simulink model "PWM_Model"  (R2019b)
settings: Solver=VariableStepAuto  StartTime=0.0  StopTime=10.0  RelTol=1e-3
model workspace (MAT data in the model file):
  MCU_freq = Simulink.Parameter
  MCU_freq.Value = 1000000
  MCU_freq.DataType = 'auto'
  MCU_freq.Dimensions = [1 1]
  MCU_timerDesiredFreq = Simulink.Parameter
  MCU_timerDesiredFreq.Value = 50
  MCU_timerDesiredFreq.DataType = 'auto'
  MCU_timerDesiredFreq.Dimensions = [1 1]
  MCU_timerPrescaler = Simulink.Parameter
  MCU_timerPrescaler.Value = 16
  MCU_timerPrescaler.DataType = 'auto'
  MCU_timerPrescaler.Dimensions = [1 1]
  Servo_PWM_0_degree = Simulink.Parameter
  Servo_PWM_0_degree.Value = 4.5
  Servo_PWM_0_degree.DataType = 'auto'
  Servo_PWM_0_degree.Dimensions = [1 1]
  Servo_PWM_180_degree = Simulink.Parameter
  Servo_PWM_180_degree.Value = 10.5
  Servo_PWM_180_degree.DataType = 'auto'
  Servo_PWM_180_degree.Dimensions = [1 1]
undefined symbols (not defined in the file): m, n, sigbuilder_block
libraries: aerolibanimutils x1
settings Model: OrderedModelArguments=off  Creator=OBU  LastModifiedBy=toons

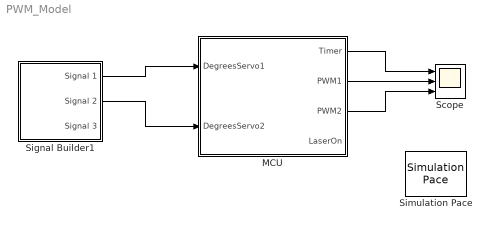
== system PWM_Model ==
  MCU : Subsystem
  Scope : Scope  NumInputPorts=3
  Signal Builder1 : Subsystem  Tag=STV Subsys  LoadFcn=sigbuilder_block('load');  StartFcn=sigbuilder_block('start');  StopFcn=sigbuilder_block('stop');  ClipboardFcn=sigbuilder_block('clipboard');  mask(Sigbuilder block){tuvar=[0:10]}
      mask help: Simulink:masks:SigbuilderBlock_MD
      mask init:
      | if ~strcmp(get_param(bdroot(gcbh),'SimulationStatus'),'stopped') tuvar = sigbuilder_block('maskInit'); end
      settings: CopyFcn=sigbuilder_block('copy');  DeleteFcn=sigbuilder_block('delete');  ModelCloseFcn=sigbuilder_block('modelClose');  PreSaveFcn=sigbuilder_block('preSave');  PauseFcn=sigbuilder_block('pause');  ContinueFcn=sigbuilder_block('continue');  NameChangeFcn=sigbuilder_block('namechange');  OpenFcn=sigbuilder_block('open',[355.2 161.4 550.8 400.2 ]);  CloseFcn=sigbuilder_block('close');
      mask Display: plot(0, 0, 100, 100,[2, 2, 32, 32, 2], [68, 8, 8, 68, 68],[32, 2], [38, 38], [32, 19, 2],[53, 60, 44], [32, 17, 17, 2],[16, 16, 31, 31]);txt = getActiveGroup(gcbh);text(2, 100, txt,'verticalAlignment', 'top');
  Simulation Pace : aerolibanimutils/Simulation Pace  SimulationPace=1  SleepMode=Auto  OutputPaceError=off  SampleTime=1/30
  wires:
  Signal Builder1/1(Signal 1) -> MCU/1("DegreesServo1 ")
  Signal Builder1/2(Signal 2) -> MCU/2(DegreesServo2)
  MCU/2("PWM1 ") -> Scope/2
  MCU/3(PWM2) -> Scope/3
  MCU/1(Timer) -> Scope/1

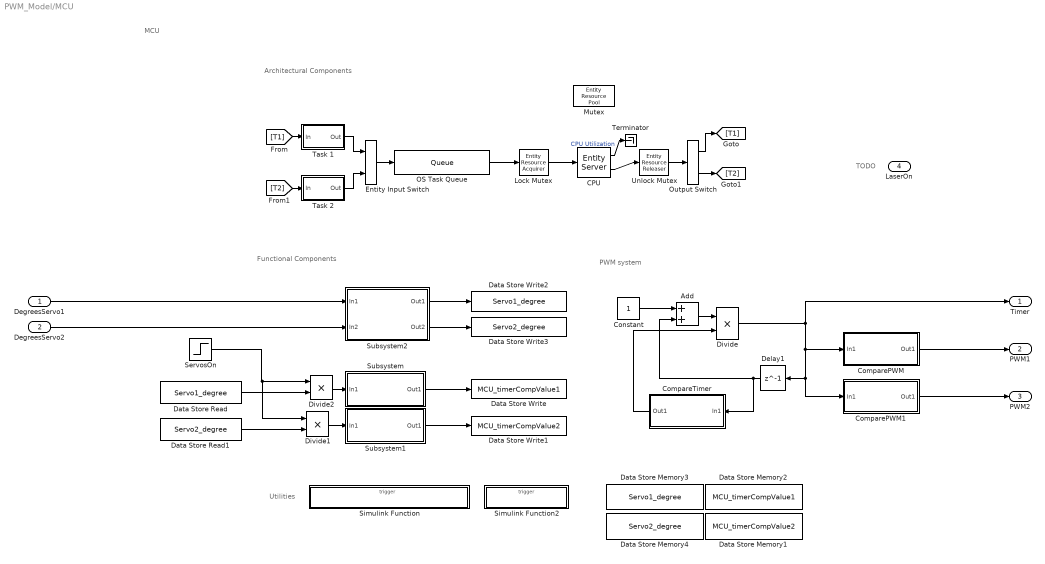
== system PWM_Model/MCU ==
  note: TODO
  note: PWM system
  note: MCU
  note: Functional Components
  note: Utilities
  note: Architectural Components
  "DegreesServo1 " : Inport
  DegreesServo2 : Inport  Port=2
  Add : Sum
  CPU : EntityServer  InputPortMessageModes=m  OutputPortMessageModes=n,m  Capacity=1  ServiceTimeSource=MATLAB action  ServiceTimeAttributeName=remExecLoad  ServiceTimeAction=dt = entity.execLoad(entity.nextSegment);  EntryAction=|  ServiceCompleteAction=|  ExitAction=|  SortingAttributeName=taskPriority  WriteResidualTimeToAttribute=on  ResidualTimeAttributeName=remExecLoad  Utilization=on
      EntryAction=|
      | start = 0;
      | entity.coreID = allocCore(start);
      | numSegments = length(entity.execLoad);
      | drawTaskTiming(entity.taskID, ...
      |                entity.nextSegment, ...
      |                numSegments, ...
      |                entity.coreID, ...
      |                entity.needsMutexForNextSegment, ...
      |                start);
      ServiceCompleteAction=|
      | switch entity.taskID
      |     case 1
      |         switch entity.nextSegment
      |             case 1
      |                 servo1_set_degree();
      |             case 2
      |                 servo2_set_degree();
      |         end
      |     case 2
      |         switch entity.nextSegment
      |             case 1
      |                 pwm1_set();
      |             case 2
      |                 pwm2_set();
      |         end
      | end
      ExitAction=|
      | complete = 1;
      | numSegments = length(entity.execLoad);
      | drawTaskTiming(entity.taskID, ...
      |                entity.nextSegment, ...
      |                numSegments, ...
      |                entity.coreID, ...
      |                entity.needsMutexForNextSegment, ...
      |                complete);
      | allocCore(entity.coreID);
      settings: OutputPortMap=o5,o9
  ComparePWM : Subsystem
  ComparePWM1 : Subsystem
  CompareTimer : Subsystem
  Constant : Constant
  Data Store Memory1 : DataStoreMemory  DataStoreName=MCU_timerCompValue2  ReadBeforeWriteMsg=warning  WriteAfterWriteMsg=warning  WriteAfterReadMsg=warning  InitialValue=400  ShowAdditionalParam=off  OutDataTypeStr=double
  Data Store Memory2 : DataStoreMemory  DataStoreName=MCU_timerCompValue1  ReadBeforeWriteMsg=warning  WriteAfterWriteMsg=warning  WriteAfterReadMsg=warning  InitialValue=400  ShowAdditionalParam=off  OutDataTypeStr=double
  Data Store Memory3 : DataStoreMemory  DataStoreName=Servo1_degree  ReadBeforeWriteMsg=warning  WriteAfterWriteMsg=warning  WriteAfterReadMsg=warning  InitialValue=400  ShowAdditionalParam=off  OutDataTypeStr=double
  Data Store Memory4 : DataStoreMemory  DataStoreName=Servo2_degree  ReadBeforeWriteMsg=warning  WriteAfterWriteMsg=warning  WriteAfterReadMsg=warning  InitialValue=400  ShowAdditionalParam=off  OutDataTypeStr=double
  Data Store Read : DataStoreRead  DataStoreName=Servo1_degree
  Data Store Read1 : DataStoreRead  DataStoreName=Servo2_degree
  Data Store Write : DataStoreWrite  DataStoreName=MCU_timerCompValue1
  Data Store Write1 : DataStoreWrite  DataStoreName=MCU_timerCompValue2
  Data Store Write2 : DataStoreWrite  DataStoreName=Servo1_degree
  Data Store Write3 : DataStoreWrite  DataStoreName=Servo2_degree
  Delay1 : Delay  DelayLength=1  SampleTime=1/(MCU_freq/MCU_timerPrescaler)
  Divide : Product  Inputs=**  SaturateOnIntegerOverflow=on  RndMeth=Zero
  Divide1 : Product  Inputs=**  SaturateOnIntegerOverflow=on  RndMeth=Zero
  Divide2 : Product  Inputs=**  SaturateOnIntegerOverflow=on  RndMeth=Zero
  Entity Input Switch : EntityInputSwitch  InputPortMessageModes=m,m  OutputPortMessageModes=m
  Lock Mutex : EntityResourceAcquirer  InputPortMessageModes=m  OutputPortMessageModes=m  EntryAction=entity.needsMutexForNextSegment = entity.needsResource(entity.nextSegment);  ResourceName=DiskLock  ResourceAmountSource=Attribute  ResourceAmount=needsMutexForNextSegment
      settings: OutputPortMap=o3
  Mutex : EntityResourcePool  ResourceName=DiskLock  ResourceAmount=1
  OS Task Queue : Queue  InputPortMessageModes=m  OutputPortMessageModes=m  Capacity=100  QueueType=Priority  PrioritySource=taskPriority  MulticastTag=TaskReady
  Output Switch : EntityOutputSwitch  InputPortMessageModes=m  OutputPortMessageModes=m,m  SwitchingCriterion=From attribute  SwitchAttributeName=taskID
  ServosOn : Step  SampleTime=0
  Simulink Function : Subsystem  TreatAsAtomicUnit=on
  Simulink Function2 : Subsystem  TreatAsAtomicUnit=on
  Subsystem : Subsystem
  Subsystem1 : Subsystem
  Subsystem2 : Subsystem
  Task 1 : Subsystem  mask{taskID=1, period=0.5, taskPriority=100, taskFunction=servo1_set_degree, servo2_set_degree, execLoad=[0.1, 0.1], needsResource=[0 0]}
      mask prompts: taskID "ID:"; taskPriority "Priority:"; taskFunction "List of runnable segments (functions):"; execLoad "Segment execution load vector:"; needsResource "Needs disk i/o resource for each segment:"
      mask DialogControl DescGroupVar Prompt: OS Task
      mask DialogControl DescTextVar Prompt: Model and simulate a task of a real-time operating system.
      mask Display: disp(['Task ' get_param(gcb, 'taskID')])
  Task 2 : Subsystem  mask{taskID=2, period=0.5, taskPriority=50, execLoad=[0.1, 0.1], taskFunction=pwm1_set,pwm2_set, needsResource=[0 0]}
      mask prompts: taskID "ID:"; taskPriority "Priority:"; execLoad "Segment execution load vector:"; taskFunction "List of runnable segments (functions):"; needsResource "Needs disk i/o resource for each segment:"
      mask DialogControl DescGroupVar Prompt: OS Task
      mask DialogControl DescTextVar Prompt: Model and simulate a task of a real-time operating system.
      mask Display: disp(['Task ' get_param(gcb, 'taskID')])
  Terminator : Terminator
  Unlock Mutex : EntityResourceReleaser  InputPortMessageModes=m  OutputPortMessageModes=m
  Timer : Outport
  "PWM1 " : Outport  Port=2
  PWM2 : Outport  Port=3
  LaserOn : Outport  Port=4
  wires:
  Task 1/1(Out) -> Entity Input Switch/1
  Divide/1 -> Timer/1, ComparePWM1/1(In1), Delay1/1, ComparePWM/1(In1)
  Entity Input Switch/1 -> OS Task Queue/1
  [T2] -> Task 2/1(In)
  Lock Mutex/1 -> CPU/1
  Task 2/1(Out) -> Entity Input Switch/2
  Output Switch/1 -> [T1]
  Unlock Mutex/1 -> Output Switch/1
  CPU/2 -> Unlock Mutex/1
  OS Task Queue/1 -> Lock Mutex/1
  Constant/1 -> Add/1
  CompareTimer/1(Out1) -> Divide/2
  Delay1/1 -> Add/2, CompareTimer/1(In1)
  Add/1 -> Divide/1
  [T1] -> Task 1/1(In)
  CPU/1 -> Terminator/1  "CPU Utilization"
  Output Switch/2 -> [T2]
  DegreesServo2/1 -> Subsystem2/2(In2)
  "DegreesServo1 "/1 -> Subsystem2/1(In1)
  ComparePWM/1(Out1) -> "PWM1 "/1
  ComparePWM1/1(Out1) -> PWM2/1
  Subsystem1/1(Out1) -> Data Store Write1/1
  Subsystem/1(Out1) -> Data Store Write/1
  Subsystem2/1(Out1) -> Data Store Write2/1
  Subsystem2/2(Out2) -> Data Store Write3/1
  Divide2/1 -> Subsystem/1(In1)
  Data Store Read/1 -> Divide2/2
  Divide1/1 -> Subsystem1/1(In1)
  ServosOn/1 -> Divide1/1, Divide2/1
  Data Store Read1/1 -> Divide1/2

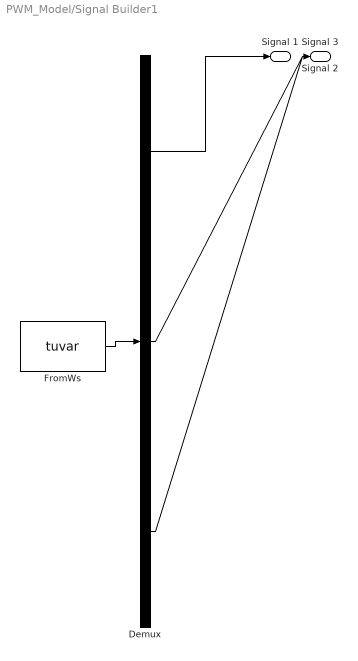
== system PWM_Model/Signal Builder1 ==
  Demux : Demux  Tag=STV Demux  Outputs=3
  FromWs : FromWorkspace  Tag=STV FromWs  VariableName=tuvar  SampleTime=0
      SigBuilderData=|
      | common.afterFinalStr = 'Extrapolate'
      | common.sampleTime = 0
      | dataSet.timeRange = [0 10]
      | dataSet.name = 'Group 1'
      | sbobj.Groups.Name = 'Group 1'
      | sbobj.Groups.Signals(1).Name = 'Signal 1'
      | sbobj.Groups.Signals(1).XData = [0 4 5 6 10]
      | sbobj.Groups.Signals(1).YData = [0 180 90 90 0]
      | sbobj.Groups.Signals(2).Name = 'Signal 2'
      | sbobj.Groups.Signals(2).XData = [0 2 5 10]
      | sbobj.Groups.Signals(2).YData = [0 0 180 180]
      | sbobj.Groups.Signals(3).Name = 'Signal 3'
      | sbobj.Groups.Signals(3).XData = [0 4 4 6 6 10]
      | sbobj.Groups.Signals(3).YData = [0 0 1 1 0 0]
  Signal 1 : Outport  Tag=STV Outport
  Signal 2 : Outport  Tag=STV Outport  Port=2
  Signal 3 : Outport  Tag=STV Outport  Port=3
  wires:
  Demux/1 -> Signal 1/1
  FromWs/1 -> Demux/1
  Demux/2 -> Signal 2/1
  Demux/3 -> Signal 3/1

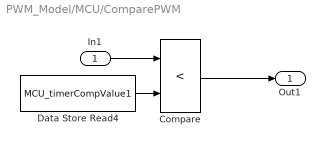
== system PWM_Model/MCU/ComparePWM ==
  In1 : Inport
  Compare : RelationalOperator  Operator=<  OutDataTypeStr=boolean  RndMeth=Nearest  InputSameDT=on
  Data Store Read4 : DataStoreRead  DataStoreName=MCU_timerCompValue1
  Out1 : Outport
  wires:
  In1/1 -> Compare/1
  Compare/1 -> Out1/1
  Data Store Read4/1 -> Compare/2

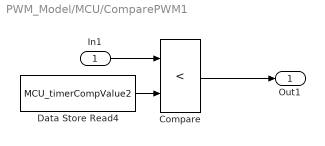
== system PWM_Model/MCU/ComparePWM1 ==
  In1 : Inport
  Compare : RelationalOperator  Operator=<  OutDataTypeStr=boolean  RndMeth=Nearest  InputSameDT=on
  Data Store Read4 : DataStoreRead  DataStoreName=MCU_timerCompValue2
  Out1 : Outport
  wires:
  In1/1 -> Compare/1
  Compare/1 -> Out1/1
  Data Store Read4/1 -> Compare/2

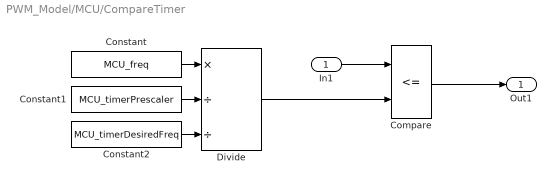
== system PWM_Model/MCU/CompareTimer ==
  In1 : Inport
  Compare : RelationalOperator  Operator=<=  OutDataTypeStr=boolean  RndMeth=Nearest  InputSameDT=on
  Constant : Constant  Value=MCU_freq
  Constant1 : Constant  Value=MCU_timerPrescaler
  Constant2 : Constant  Value=MCU_timerDesiredFreq
  Divide : Product  Inputs=*//
  Out1 : Outport
  wires:
  Compare/1 -> Out1/1
  Constant2/1 -> Divide/3
  Constant1/1 -> Divide/2
  Constant/1 -> Divide/1
  Divide/1 -> Compare/2
  In1/1 -> Compare/1

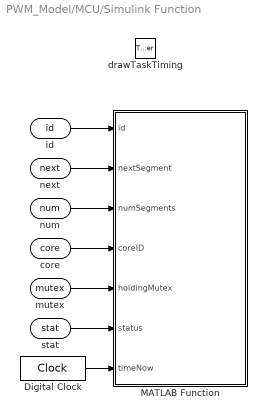
== system PWM_Model/MCU/Simulink Function ==
  drawTaskTiming : TriggerPort  TriggerType=function-call  IsSimulinkFunction=on  FunctionName=drawTaskTiming  VariantControl=Variant
  Digital Clock : DigitalClock  SampleTime=-1
  MATLAB Function : MATLAB Function  TreatAsAtomicUnit=on
  id : ArgIn  DisableCoverage=on  ArgumentName=id
  next : ArgIn  Port=2  ArgumentName=next
  num : ArgIn  Port=3  ArgumentName=num
  core : ArgIn  Port=4  ArgumentName=core
  mutex : ArgIn  Port=5  ArgumentName=mutex
  stat : ArgIn  Port=6  ArgumentName=stat
  wires:
  id/1 -> MATLAB Function/1(id)
  next/1 -> MATLAB Function/2(nextSegment)
  num/1 -> MATLAB Function/3(numSegments)
  Digital Clock/1 -> MATLAB Function/7(timeNow)
  core/1 -> MATLAB Function/4(coreID)
  mutex/1 -> MATLAB Function/5(holdingMutex)
  stat/1 -> MATLAB Function/6(status)

== system PWM_Model/MCU/Simulink Function2 ==
  allocCore : TriggerPort  TriggerType=function-call  IsSimulinkFunction=on  FunctionName=allocCore  VariantControl=Variant
  MATLAB Function : MATLAB Function  TreatAsAtomicUnit=on
  status : ArgIn  ArgumentName=status
  id : ArgOut  ArgumentName=id
  wires:
  status/1 -> MATLAB Function/1(status)
  MATLAB Function/1(id) -> id/1

== system PWM_Model/MCU/Subsystem ==
  In1 : Inport
  Subsystem : Subsystem
  Out1 : Outport
  wires:
  In1/1 -> Subsystem/1(In1)
  Subsystem/1(Out1) -> Out1/1

== system PWM_Model/MCU/Subsystem1 ==
  In1 : Inport
  Subsystem : Subsystem
  Out1 : Outport
  wires:
  In1/1 -> Subsystem/1(In1)
  Subsystem/1(Out1) -> Out1/1

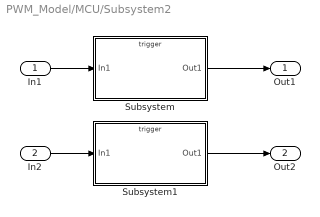
== system PWM_Model/MCU/Subsystem2 ==
  In1 : Inport
  In2 : Inport  Port=2
  Subsystem : Subsystem
  Subsystem1 : Subsystem
  Out1 : Outport
  Out2 : Outport  Port=2
  wires:
  In1/1 -> Subsystem/1(In1)
  Subsystem/1(Out1) -> Out1/1
  Subsystem1/1(Out1) -> Out2/1
  In2/1 -> Subsystem1/1(In1)

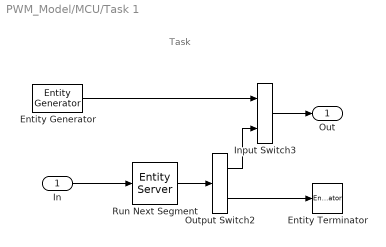
== system PWM_Model/MCU/Task 1 ==
  note: Task
  In : Inport
  Entity Generator : EntityGenerator  OutputPortMessageModes=m  Period=period  AttributeName=period|numSegments|execLoad|taskPriority|taskID|nextSegment|complete|coreID|needsMutexForNextSegment|needsResource  AttributeInitialValue=period|length(execLoad)|[execLoad zeros(1,20-length(execLoad))]|taskPriority|taskID|1|1|-1|0|[needsResource zeros(1,100-length(needsResource))]  EntityType=Structured  EntityTypeName=Task  EntityPriority=taskPriority
  Entity Terminator : EntityTerminator  InputPortMessageModes=m
  Input Switch3 : EntityInputSwitch  InputPortMessageModes=m,m  OutputPortMessageModes=m
  Output Switch2 : EntityOutputSwitch  InputPortMessageModes=m  OutputPortMessageModes=m,m  SwitchingCriterion=From attribute  SwitchAttributeName=complete
  Run Next Segment : EntityServer  InputPortMessageModes=m  OutputPortMessageModes=m  Capacity=1  ServiceTimeValue=0  ServiceCompleteAction=|
      | entity.nextSegment=entity.nextSegment+1;
      | if entity.nextSegment>entity.numSegments
      |     entity.complete=2;
      | else
      |     entity.needsMutexForNextSegment=entity.needsResource(entity.nextSegment);
      | end
  Out : Outport  VectorParamsAs1DForOutWhenUnconnected=off
  wires:
  In/1 -> Run Next Segment/1
  Entity Generator/1 -> Input Switch3/1
  Input Switch3/1 -> Out/1
  Run Next Segment/1 -> Output Switch2/1
  Output Switch2/1 -> Input Switch3/2
  Output Switch2/2 -> Entity Terminator/1

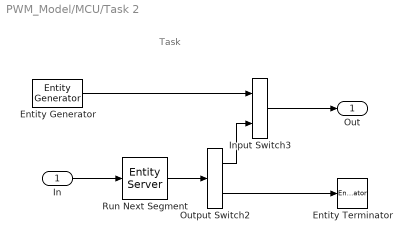
== system PWM_Model/MCU/Task 2 ==
  note: Task
  In : Inport
  Entity Generator : EntityGenerator  OutputPortMessageModes=m  Period=period  AttributeName=period|numSegments|execLoad|taskPriority|taskID|nextSegment|complete|coreID|needsMutexForNextSegment|needsResource  AttributeInitialValue=period|length(execLoad)|[execLoad zeros(1,20-length(execLoad))]|taskPriority|taskID|1|1|-1|0|[needsResource zeros(1,100-length(needsResource))]  EntityType=Structured  EntityTypeName=Task  EntityPriority=taskPriority
  Entity Terminator : EntityTerminator  InputPortMessageModes=m
  Input Switch3 : EntityInputSwitch  InputPortMessageModes=m,m  OutputPortMessageModes=m
  Output Switch2 : EntityOutputSwitch  InputPortMessageModes=m  OutputPortMessageModes=m,m  SwitchingCriterion=From attribute  SwitchAttributeName=complete
  Run Next Segment : EntityServer  InputPortMessageModes=m  OutputPortMessageModes=m  Capacity=1  ServiceTimeValue=0  ServiceCompleteAction=|
      | entity.nextSegment=entity.nextSegment+1;
      | if entity.nextSegment>entity.numSegments
      |     entity.complete=2;
      | else
      |     entity.needsMutexForNextSegment=entity.needsResource(entity.nextSegment);    
      | end
  Out : Outport  VectorParamsAs1DForOutWhenUnconnected=off
  wires:
  In/1 -> Run Next Segment/1
  Entity Generator/1 -> Input Switch3/1
  Input Switch3/1 -> Out/1
  Run Next Segment/1 -> Output Switch2/1
  Output Switch2/1 -> Input Switch3/2
  Output Switch2/2 -> Entity Terminator/1

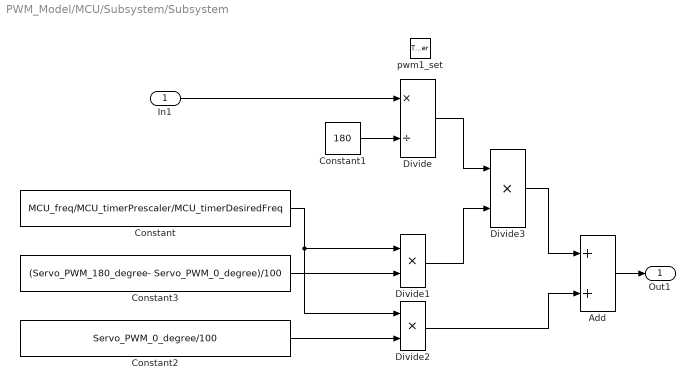
== system PWM_Model/MCU/Subsystem/Subsystem ==
  In1 : Inport
  pwm1_set : TriggerPort  TriggerType=function-call  IsSimulinkFunction=on  FunctionName=pwm1_set  VariantControl=Variant
  Add : Sum
  Constant : Constant  Value=MCU_freq/MCU_timerPrescaler/MCU_timerDesiredFreq
  Constant1 : Constant  Value=180
  Constant2 : Constant  Value=Servo_PWM_0_degree/100
  Constant3 : Constant  Value=(Servo_PWM_180_degree- Servo_PWM_0_degree)/100
  Divide : Product  Inputs=*/  SaturateOnIntegerOverflow=on  RndMeth=Zero
  Divide1 : Product  Inputs=**  SaturateOnIntegerOverflow=on  RndMeth=Zero
  Divide2 : Product  Inputs=**  SaturateOnIntegerOverflow=on  RndMeth=Zero
  Divide3 : Product  Inputs=**  SaturateOnIntegerOverflow=on  RndMeth=Zero
  Out1 : Outport
  wires:
  Constant1/1 -> Divide/2
  Constant/1 -> Divide1/1, Divide2/1
  Constant2/1 -> Divide2/2
  Constant3/1 -> Divide1/2
  Divide/1 -> Divide3/1
  Divide1/1 -> Divide3/2
  Divide2/1 -> Add/2
  Divide3/1 -> Add/1
  In1/1 -> Divide/1
  Add/1 -> Out1/1

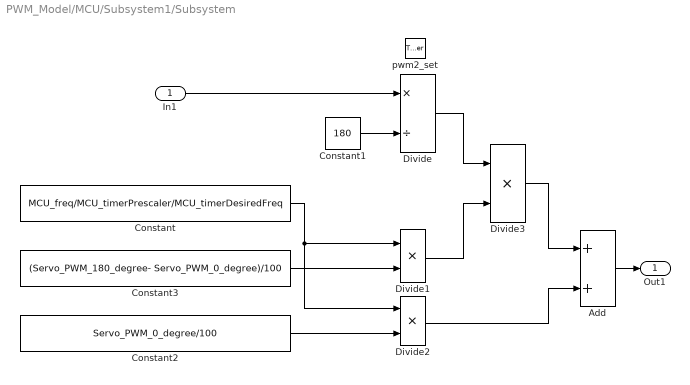
== system PWM_Model/MCU/Subsystem1/Subsystem ==
  In1 : Inport
  pwm2_set : TriggerPort  TriggerType=function-call  IsSimulinkFunction=on  FunctionName=pwm2_set  VariantControl=Variant
  Add : Sum
  Constant : Constant  Value=MCU_freq/MCU_timerPrescaler/MCU_timerDesiredFreq
  Constant1 : Constant  Value=180
  Constant2 : Constant  Value=Servo_PWM_0_degree/100
  Constant3 : Constant  Value=(Servo_PWM_180_degree- Servo_PWM_0_degree)/100
  Divide : Product  Inputs=*/  SaturateOnIntegerOverflow=on  RndMeth=Zero
  Divide1 : Product  Inputs=**  SaturateOnIntegerOverflow=on  RndMeth=Zero
  Divide2 : Product  Inputs=**  SaturateOnIntegerOverflow=on  RndMeth=Zero
  Divide3 : Product  Inputs=**  SaturateOnIntegerOverflow=on  RndMeth=Zero
  Out1 : Outport
  wires:
  Constant1/1 -> Divide/2
  Constant3/1 -> Divide1/2
  Divide2/1 -> Add/2
  Divide/1 -> Divide3/1
  In1/1 -> Divide/1
  Constant/1 -> Divide1/1, Divide2/1
  Add/1 -> Out1/1
  Constant2/1 -> Divide2/2
  Divide3/1 -> Add/1
  Divide1/1 -> Divide3/2

== system PWM_Model/MCU/Subsystem2/Subsystem ==
  In1 : Inport
  servo1_set_degree : TriggerPort  TriggerType=function-call  IsSimulinkFunction=on  FunctionName=servo1_set_degree  VariantControl=Variant
  Out1 : Outport
  wires:
  In1/1 -> Out1/1

== system PWM_Model/MCU/Subsystem2/Subsystem1 ==
  In1 : Inport
  servo2_set_degree : TriggerPort  TriggerType=function-call  IsSimulinkFunction=on  FunctionName=servo2_set_degree  VariantControl=Variant
  Out1 : Outport
  wires:
  In1/1 -> Out1/1

== matlab function PWM_Model/MCU/Simulink Function2/MATLAB Function ==
  data: status input; id output
function id = allocCore(status)
%#codegen

persistent allocCores
if isempty(allocCores)
    allocCores = zeros(1,100);
end

id = -1;

if status == 0
    for i = 1:100
        if allocCores(i) == 0
            id = i;
            allocCores(i) = 1;
            break;
        end
    end
else
    allocCores(status) = 0;
end

== matlab function PWM_Model/MCU/Simulink Function/MATLAB Function ==
  data: id input; nextSegment input; numSegments input; coreID input; holdingMutex input; status input; timeNow input
function fcn(id, nextSegment, numSegments, coreID, holdingMutex, status, timeNow)
%#codegen

persistent ax lastTime

cBlue = [18/255 104/255 179/255];
cRed = [237/255 36/255 38/255];
cGreen = [155 190 61]/255;
allColors = [cBlue; cRed; cGreen];

coder.extrinsic('evalin');
numCores = 2;
numTasks = 2;
mutexY = numCores+1;

if isempty(ax)
    close all;
    fig = figure('position',[762 173 920 326]);
    ax = axes;
    set(ax,'box','on');
    grid on; hold on;
    set(ax,'XLim',[0 20],'YLim',[0 numCores+1+1],'YTick',1:numCores+1,'xminorgrid','on');
    set(fig,'name','Task Timing');
    
    lastTime = zeros(1,numTasks)-1;
end

thisColor = allColors(id,:);
mutexColor = allColors(3,:);
coder.extrinsic('num2str');
switch status
    case 0
        % Task is entering CPU
        lastTime(id) = timeNow;        
    case 1
        % Task is exiting CPU - segment complete
        rectangle('parent', ax, ...
            'position', [lastTime(id), coreID-0.3, timeNow-lastTime(id), 0.6], ...
            'facecolor', thisColor, 'edgecolor', [0 0 0]);
        if holdingMutex
            rectangle('parent', ax, ...
                'position', [lastTime(id), mutexY-0.3, timeNow-lastTime(id), 0.6], ...
                'facecolor', mutexColor, 'edgecolor', [0 0 0]);        
        end
end
